simulink model "simulink_miniproyectoRE"  (R2023b)
settings: Solver=VariableStepAuto  StartTime=0.0  StopTime=50  RelTol=1e-3
undefined symbols (not defined in the file): A_eval, B_eval, K
settings Model: Creator=yonathan  LastModifiedBy=yonathan

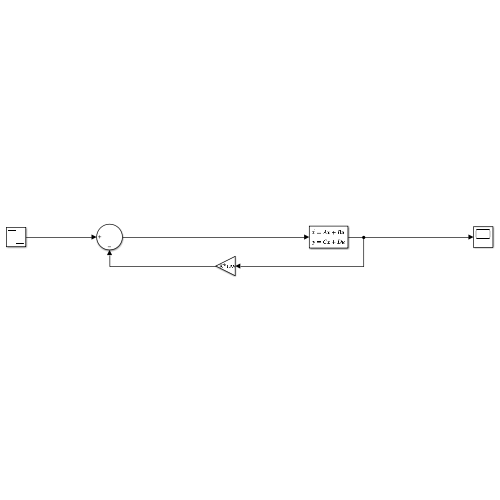
[thumbnail: Simulink's stored preview of the top-level diagram]
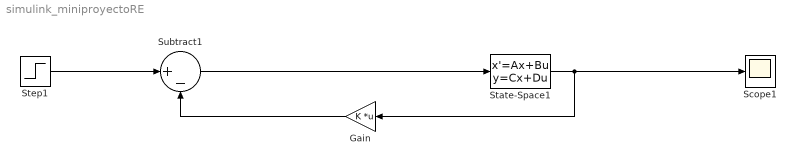
== system simulink_miniproyectoRE ==
  Gain : Gain  Gain=K  Multiplication=Matrix(K*u) (u vector)
  Scope1 : Scope
  State-Space1 : StateSpace  A=A_eval  B=B_eval  C=eye(6)  D=zeros(6,1)  InitialCondition=[0 0 0 0 0.05 0]
  Step1 : Step  Before=0.05  After=0  SampleTime=0
  Subtract1 : Sum  Inputs=|+-
  wires:
  State-Space1/1 -> Gain/1, Scope1/1
  Subtract1/1 -> State-Space1/1
  Step1/1 -> Subtract1/1
  Gain/1 -> Subtract1/2
